simulink model "DDMvsIDM"  (Simulink 7.8)
settings: Solver=ode45  StartTime=0.0  StopTime=10.0  RelTol=1e-3
settings Model: Creator=Administrator  LastModifiedBy=Administrator

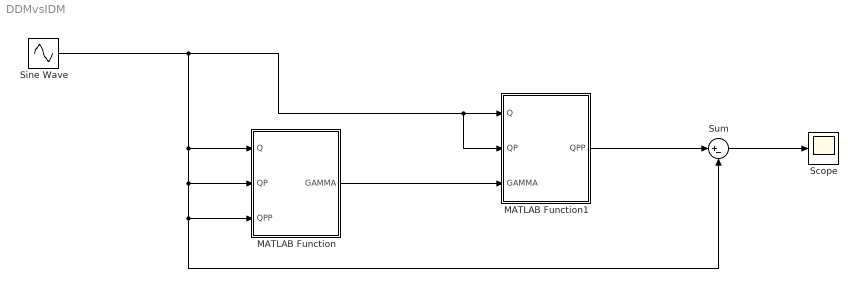
== system DDMvsIDM ==
  MATLAB Function : MATLAB Function  TreatAsAtomicUnit=on
  MATLAB Function1 : MATLAB Function  TreatAsAtomicUnit=on
  Scope : Scope
  Sine Wave : Sin  Amplitude=[0.1;0.2]  Frequency=20  SampleTime=0
  Sum : Sum  Inputs=|+-
  wires:
  MATLAB Function/1(GAMMA) -> MATLAB Function1/3(GAMMA)
  Sine Wave/1 -> MATLAB Function1/1(Q), MATLAB Function1/2(QP), MATLAB Function/1(Q), MATLAB Function/2(QP), MATLAB Function/3(QPP), Sum/2
  MATLAB Function1/1(QPP) -> Sum/1
  Sum/1 -> Scope/1

== matlab function MATLAB Function1 ==
  data: Q input double size=[2 1]; QP input double size=[2 1]; GAMMA input double size=[2 1]; QPP output double size=[2 1]
function QPP = fcn2(Q,QP,GAMMA)
%#codegen
L1 = 0.2;       % m
L2 = 0.1442;    % m
M2 = 0.464;     % kg
ZZ1 = 0.0045;
ZZ2 = 0.0015;
MX2 = 0.0257;
MY2 = 0;
QPP1 = GAMMA(1)*(ZZ1 + ZZ2 + L1^2*M2 + 2*L1*MX2*cos(Q(1)) ...
    - 2*L1*MY2*sin(Q(1))) - QP(2)*(QP(1)*(L1*MY2*cos(Q(1)) ...
    + L1*MX2*sin(Q(1))) + QP(2)*(L1*MY2*cos(Q(1)) + L1*MX2*sin(Q(1)))) ...
    + GAMMA(2)*(ZZ2 + L1*MX2*cos(Q(1)) - L1*MY2*sin(Q(1))) ...
    - QP(1)*QP(2)*(L1*MY2*cos(Q(1)) + L1*MX2*sin(Q(1)));
QPP2 = (L1*MY2*cos(Q(1)) + L1*MX2*sin(Q(1)))*QP(1)^2 + GAMMA(2)*ZZ2 ...
    + GAMMA(1)*(ZZ2 + L1*MX2*cos(Q(1)) - L1*MY2*sin(Q(1)));
QPP = [QPP1
       QPP2];

== matlab function MATLAB Function ==
  data: Q input double size=[2 1]; GAMMA output double size=[2 1]; QP input double size=[2 1]; QPP input double size=[2 1]
function GAMMA = fcn1(Q,QP,QPP)
%#codegen
L1 = 0.2;       % m
L2 = 0.1442;    % m
M2 = 0.464;     % kg
ZZ1 = 0.0045;
ZZ2 = 0.0015;
MX2 = 0.0257;
MY2 = 0;
GAMMA1 = QPP(1)*(ZZ1 + ZZ2 + L1^2*M2 + 2*L1*MX2*cos(Q(1)) - 2*L1*MY2*sin(Q(1))) ...
    - QP(2)*(QP(1)*(L1*MY2*cos(Q(1)) + L1*MX2*sin(Q(1))) + QP(2)*(L1*MY2*cos(Q(1)) ...
    + L1*MX2*sin(Q(1)))) + QPP(2)*(ZZ2 + L1*MX2*cos(Q(1)) - L1*MY2*sin(Q(1))) ...
    - QP(1)*QP(2)*(L1*MY2*cos(Q(1)) + L1*MX2*sin(Q(1)));
GAMMA2 = (L1*MY2*cos(Q(1)) + L1*MX2*sin(Q(1)))*QP(1)^2 + QPP(2)*ZZ2 ...
    + QPP(1)*(ZZ2 + L1*MX2*cos(Q(1)) - L1*MY2*sin(Q(1)));
GAMMA = [GAMMA1
         GAMMA2];
